simulink model "TestPerturacionesReferenciaP"  (R2021b)
settings: Solver=VariableStepAuto  StartTime=0.0  StopTime=20  RelTol=1e-3
libraries: cstblocks x5
settings Model: Creator=JUAN DAVID  LastModifiedBy=parra
settings SolverCC: AlgebraicLoopSolver=TrustRegion
settings DataIOCC: ReturnWorkspaceOutputs=off
settings DebuggingCC: ArithmeticOperatorsInVariantConditions=warning
settings SFSimCC: CustomCodeUndefinedFunction=UseInterfaceOnly
settings RTWCC: DLArmComputeVersion=20.02.1

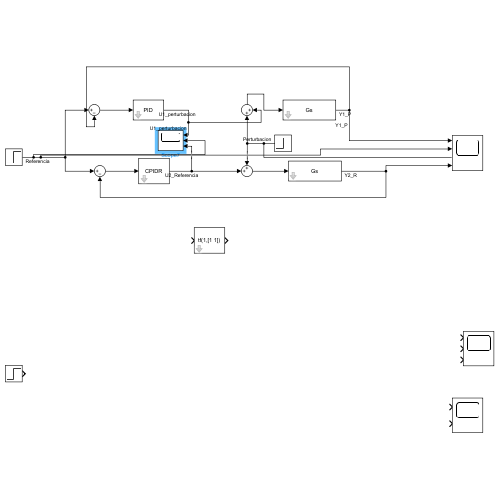
[thumbnail: Simulink's stored preview of the top-level diagram]
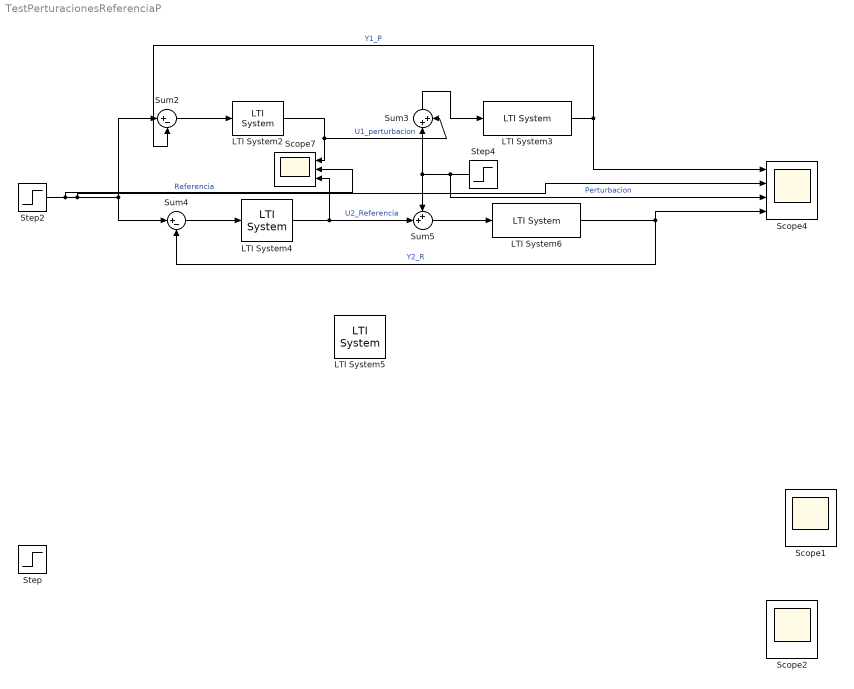
== system TestPerturacionesReferenciaP ==
  LTI System2 : cstblocks/LTI System  sys=PID  IC=[]
  LTI System3 : cstblocks/LTI System  sys=Gs  IC=[]
  LTI System4 : cstblocks/LTI System  sys=CPIDR  IC=[]
  LTI System5 : cstblocks/LTI System  sys=tf(1,[1 1])  IC=[]
  LTI System6 : cstblocks/LTI System  sys=Gs  IC=[]
  Scope1 : Scope  NumInputPorts=3
  Scope2 : Scope  NumInputPorts=2
  Scope4 : Scope  NumInputPorts=4
  Scope7 : Scope  NumInputPorts=3
  Step : Step  SampleTime=0
  Step2 : Step  After=2  SampleTime=0
  Step4 : Step  Time=1.2  SampleTime=0
  Sum2 : Sum  Inputs=|+-
  Sum3 : Sum  Inputs=|++
  Sum4 : Sum  Inputs=|+-
  Sum5 : Sum  Inputs=++|
  wires:
  Step2/1 -> Scope7/2, Scope4/2, Sum4/1, Sum2/1  "Referencia"
  LTI System2/1 -> Scope7/1, Sum3/2  "U1_perturbacion"
  Sum3/1 -> LTI System3/1
  Sum2/1 -> LTI System2/1
  Sum4/1 -> LTI System4/1
  LTI System4/1 -> Scope7/3, Sum5/2  "U2_Referencia"
  Step4/1 -> Scope4/3, Sum5/1, Sum3/1  "Perturbacion"
  Sum5/1 -> LTI System6/1
  LTI System3/1 -> Scope4/1, Sum2/2  "Y1_P"
  LTI System6/1 -> Scope4/4, Sum4/2  "Y2_R"
